simulink model "T3"  (R2015a)
settings: Solver=ode45  StartTime=0.0  StopTime=10.0  RelTol=1e-3
settings Model: Creator=Benjamin Nicolas  LastModifiedBy=Benjamin Nicolas

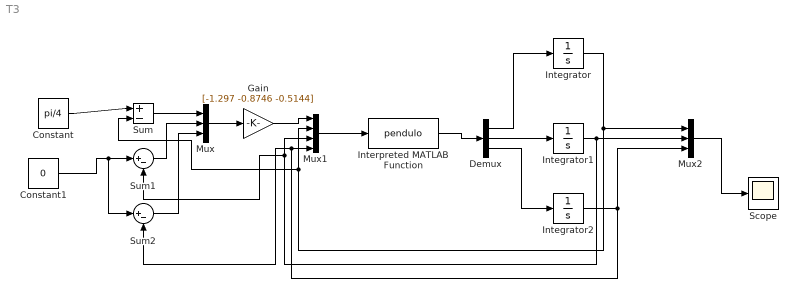
== system T3 ==
  Constant : Constant  Value=pi/4
  Constant1 : Constant  Value=0
  Demux : Demux  Outputs=3
  Gain : Gain  Gain=[-1.297 -0.8746 -0.5144]
  Integrator : Integrator
  Integrator1 : Integrator
  Integrator2 : Integrator
  Interpreted MATLAB Function : MATLABFcn  MATLABFcn=pendulo
  Mux : Mux  Inputs=3
  Mux1 : Mux
  Mux2 : Mux  Inputs=3
  Scope : Scope
  Sum : Sum  Inputs=|+-
  Sum1 : Sum  Inputs=|+-
  Sum2 : Sum  Inputs=|+-
  wires:
  Sum2/1 -> Mux/3
  Sum1/1 -> Mux/2
  Sum/1 -> Mux/1
  Mux/1 -> Gain/1
  Gain/1 -> Mux1/1
  Mux1/1 -> Interpreted MATLAB Function/1
  Interpreted MATLAB Function/1 -> Demux/1
  Demux/1 -> Integrator/1
  Demux/2 -> Integrator1/1
  Demux/3 -> Integrator2/1
  Integrator/1 -> Mux2/1, Mux1/2, Sum/2
  Integrator1/1 -> Mux2/2, Mux1/3, Sum1/2
  Integrator2/1 -> Mux1/4, Sum2/2, Mux2/3
  Constant1/1 -> Sum2/1, Sum1/1
  Constant/1 -> Sum/1
  Mux2/1 -> Scope/1
